simulink model "Fault_Estimator"  (R2023a)
settings: Solver=VariableStepAuto  StartTime=0.0  StopTime=60  RelTol=1e-3
values from neighbouring files (symbols this model uses):
  A = [O_As zeros(n,s)]    [Adaptive_Ka_Test.m]    (also in Fault_Estimator_Parameters.mat = [0.999941069129  7.16658673766e-07  5.87954926208e-05  0; -1; UIO_Calculation.m)
  A_bar = G*A    [Adaptive_Ka_Test.m]    (also in Fault_Estimator_Parameters.mat = [0 -1.34709716077e-07 5.89016941685e-05 -5.89016941685e-05 0; UIO_Calculation.m)
  A_zero = O_Az    [Adaptive_Ka_Test.m]    (also in Fault_Estimator_Parameters.mat = [0.00133629303608 -0.0295574271846 0.028990279103 0.00138410; LPV_Time_Varient_Parameter.m; UIO_Calculation.m)
  B = O_B    [Adaptive_Ka_Test.m]    (also in Fault_Estimator_Parameters.mat = [6.48267970563e-05  3.7353807763e-08; 6.66149393921e-09  6.4; LPV_Time_Varient_Parameter.m; UIO_Calculation.m)
  B_bar = G*B    [Adaptive_Ka_Test.m]    (also in Fault_Estimator_Parameters.mat = [0  0; 6.66149393921e-09  6.48911324748e-05; 6.63859792846e-; UIO_Calculation.m)
  C = [C_star F]    [Adaptive_Ka_Test.m]    (also in Fault_Estimator_Parameters.mat = [1  0  0  0; 0  1  0  0; 0  0  1  1]; UIO_Calculation.m)
  D = [1/154;0;0]    [Adaptive_Ka_Test.m]    (also in UIO_Calculation.m)
  E_zero = O_E*E    [Adaptive_Ka_Test.m]    (also in Fault_Estimator_Parameters.mat = [0.000413364504327 -0.000387576328554 -0.000192232694 -0.013; UIO_Calculation.m)
  G = T-T*D*H*C*T    [Adaptive_Ka_Test.m]    (also in Fault_Estimator_Parameters.mat = [0  0  0; 0  1  0; 0  0  1; 0  0  -1]; UIO_Calculation.m)
  H = inv(transpose(C*T*D)*C*T*D)*transpose(C*T*D)    [Adaptive_Ka_Test.m]    (also in Fault_Estimator_Parameters.mat = [154 0 0]; UIO_Calculation.m)
  Ka = inv(value(U))*value(N_bar)    [Adaptive_Ka_Test.m]    (also in Fault_Estimator_Parameters.mat = [-1.05152228748e-07  -0.00319474208396  -2.37139603589e-10; ; Ka.mat = [0.202280164209  0.202279756548  0.594992063891; 0.202157428; UIO_Calculation.m)
  L_bar = (N-T*D*H*C*N+T*D*H)    [Adaptive_Ka_Test.m]    (also in Fault_Estimator_Parameters.mat = [1  0  0; 0  0  0; 0  0  0; 0  0  1]; UIO_Calculation.m)
  N = temp(1:n+s,n+1:n+p)    [Adaptive_Ka_Test.m]    (also in Fault_Estimator_Parameters.mat = [0  0  0; 0  0  0; 0  0  0; 0  0  1]; UIO_Calculation.m)
  p = 3    [Adaptive_Ka_Test.m]    (also in Fault_Estimator_Parameters.mat; UIO_Calculation.m; test.m = plot(transpose(Xt_hat)-transpose(Xt(:,t+1:t+6000))))
  T = temp(1:n+s,1:n)    [Adaptive_Ka_Test.m]    (also in Fault_Estimator_Parameters.mat = [1  0  0; 0  1  0; 0  0  1; 0  0  -1]; UIO_Calculation.m)
libraries: simulink x2
settings Model: Creator=sepeh  LastModifiedBy=sepeh

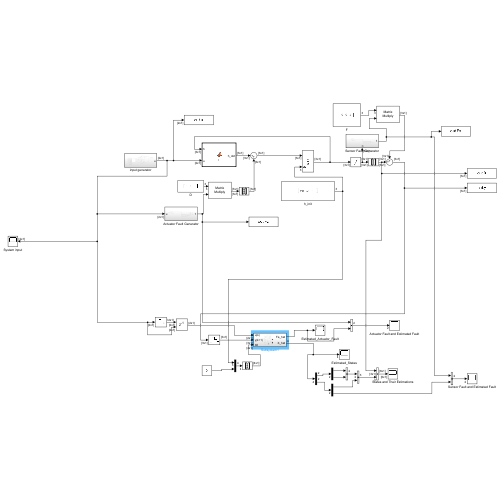
[thumbnail: Simulink's stored preview of the top-level diagram]
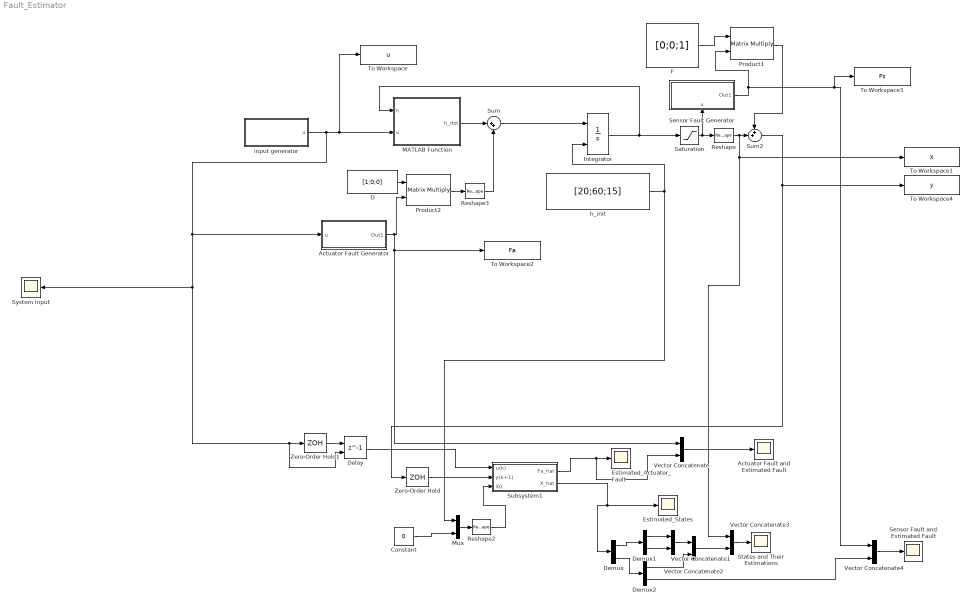
== system Fault_Estimator ==
  Actuator Fault Generator : Subsystem
  Actuator Fault and Estimated Fault : Scope
  Constant : Constant  Value=0
  D : Constant  Value=[1;0;0]
  Delay : Delay  DelayLength=1  InitialConditionSource=Input port  InitialCondition=0  SampleTime=0.01
      settings: InputPortMap=u0,p4
  Demux : Demux  Outputs=2
  Demux1 : Demux  Outputs=2
  Demux2 : Demux  Outputs=2
  Estimated_Actuator_Fault : Scope
  Estimated_States : Scope
  F : Constant  Value=[0;0;1]
  Integrator : Integrator  InitialConditionSource=external
  MATLAB Function : MATLAB Function  TreatAsAtomicUnit=on
  Mux : Mux  Inputs=2
  Product1 : Product  Multiplication=Matrix(*)
  Product2 : Product  Multiplication=Matrix(*)
  Reshape : Reshape  OutputDimensionality=Column vector (2-D)
  Reshape2 : Reshape  OutputDimensionality=Column vector (2-D)
  Reshape3 : Reshape  OutputDimensionality=Column vector (2-D)
  Saturation : Saturate  UpperLimit=100  LowerLimit=0
  Sensor Fault Generator : Subsystem
      settings: PortSchema="{\"entries\":[{\"content\":{\"sides\":[{\"content\":{},\"type\":\"ConnectorPlacement.EquallySpacedRectSide\",\"uuid\":\"8737017c-7270-4c54-a415-3a022d708922\"},{\"content\":{\"connectorIds\":[\"Out1\"],\"side\":\"RIGHT\"},\"type\":\"ConnectorPlacement.EquallySpacedRectSide\",\"uuid\":\"227575ae-1db5-4c8b-a626-16b54a509aa1\"},{\"content\":{\"side\":\"TOP\"},\"type\":\"ConnectorPlacement.EquallySpacedRectSide\",\"uuid\":\"ce2fa024-2e15-4882-8a20-94458726743e\"},{\"content\":{\"connectorIds\":[\"In1\"],\"side\":\"BOTTOM\"},\"type\":\"ConnectorPlacement.EquallySpacedRectSide\",\"uuid\":\"c4ae589d-782a-4398-85fd-5b05ba97c294\"}]},\"type\":\"ConnectorPlacement.EquallySpacedConnector\",\"uuid\":\"70d82ebf-b199-4a7a-86b9-c10264c6c64d\"}],\"packageUris\":[\"http://schema.mathworks.com/mf0/Connector/R2020b\"],\"version\":\"1.0\"}"
  Sensor Fault and Estimated Fault : Scope
  States and Their Estimations : Scope
  Subsystem1 : Subsystem
  Sum : Sum  Inputs=|++
  Sum2 : Sum  Inputs=++|
  System input : Scope
  To Workspace : ToWorkspace  VariableName=u  SaveFormat=Timeseries  SampleTime=0.01
  To Workspace1 : ToWorkspace  VariableName=X  SaveFormat=Timeseries  SampleTime=0.01
  To Workspace2 : ToWorkspace  VariableName=Fa  SaveFormat=Timeseries  SampleTime=0.01
  To Workspace3 : ToWorkspace  VariableName=Fs  SaveFormat=Timeseries  SampleTime=0.01
  To Workspace4 : ToWorkspace  VariableName=y  SaveFormat=Timeseries  SampleTime=0.01
  Vector Concatenate{,1..4} (5 alike) : Concatenate
  Zero-Order Hold : ZeroOrderHold  SampleTime=0.01
  Zero-Order Hold1 : ZeroOrderHold  SampleTime=0.01
  h_init : Constant  Value=[20;60;15]
  input generator : Subsystem
  wires:
  Integrator/1 -> Saturation/1, MATLAB Function/1(h)
  Zero-Order Hold1/1 -> Delay/1
  Delay/1 -> Subsystem1/1(u(k))
  Zero-Order Hold/1 -> Subsystem1/2(y(k+1))
  Sum2/1 -> To Workspace4/1, Zero-Order Hold/1
  input generator/1(u) -> To Workspace/1, MATLAB Function/2(u), Actuator Fault Generator/1(u), Delay/2, Zero-Order Hold1/1, System input/1
  MATLAB Function/1(h_dot) -> Sum/1
  Sum/1 -> Integrator/1
  Subsystem1/2(X_hat) -> Estimated_States/1, Demux/1
  Subsystem1/1(Fa_hat) -> Vector Concatenate/2, Estimated_Actuator_Fault/1
  Vector Concatenate/1 -> Actuator Fault and Estimated Fault/1
  h_init/1 -> Mux/1, Integrator/2
  F/1 -> Product1/1
  Saturation/1 -> Reshape/1, Sensor Fault Generator/1(u)
  Reshape/1 -> To Workspace1/1, Vector Concatenate3/1, Sum2/2
  Product1/1 -> Sum2/1
  Constant/1 -> Mux/2
  Mux/1 -> Reshape2/1
  Reshape2/1 -> Subsystem1/3(X0)
  D/1 -> Product2/1
  Reshape3/1 -> Sum/2
  Product2/1 -> Reshape3/1
  Demux/1 -> Demux1/1
  Demux/2 -> Demux2/1
  Demux1/1 -> Vector Concatenate1/1
  Demux1/2 -> Vector Concatenate1/2
  Vector Concatenate1/1 -> Vector Concatenate2/1
  Demux2/1 -> Vector Concatenate2/2
  Vector Concatenate2/1 -> Vector Concatenate3/2
  Vector Concatenate3/1 -> States and Their Estimations/1
  Demux2/2 -> Vector Concatenate4/2
  Actuator Fault Generator/1(Out1) -> To Workspace2/1, Vector Concatenate/1, Product2/2
  Vector Concatenate4/1 -> Sensor Fault and Estimated Fault/1
  Sensor Fault Generator/1(Out1) -> Product1/2, To Workspace3/1, Vector Concatenate4/1

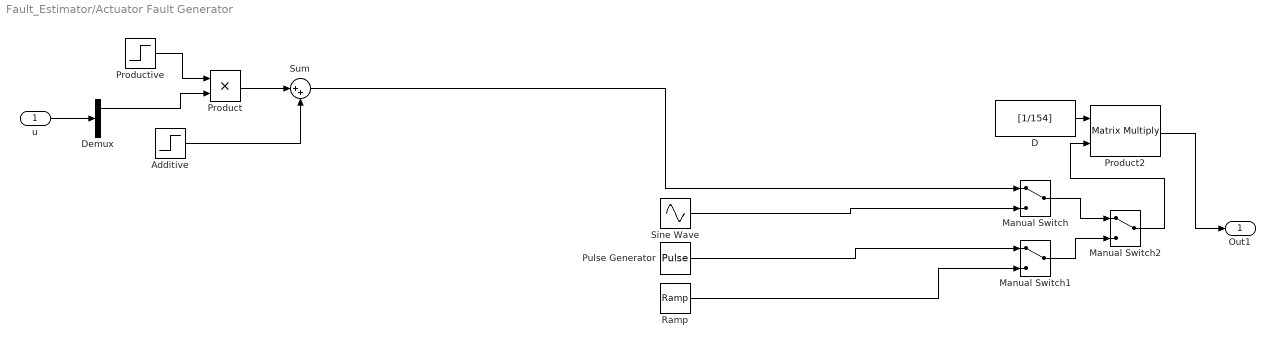
== system Fault_Estimator/Actuator Fault Generator ==
  u : Inport
  Additive : Step  Time=20  After=-10  SampleTime=0
  D : Constant  Value=[1/154]
  Demux : Demux  Outputs=2
  Manual Switch : ManualSwitch
  Manual Switch1 : ManualSwitch
  Manual Switch2 : ManualSwitch
  Product : Product
  Product2 : Product  Multiplication=Matrix(*)
  Productive : Step  Time=20  After=-0.2  SampleTime=0
  Pulse Generator : DiscretePulseGenerator  PulseType=Time based  Amplitude=-100  Period=10  PulseWidth=50
  Ramp : simulink/Sources/Ramp  slope=-10  start=30  InitialOutput=0
  Sine Wave : Sin  Amplitude=50  Bias=-100  SampleTime=0
  Sum : Sum  Inputs=|++
  Out1 : Outport
  wires:
  Manual Switch1/1 -> Manual Switch2/2
  Manual Switch/1 -> Manual Switch2/1
  u/1 -> Demux/1
  Demux/1 -> Product/2
  Product/1 -> Sum/1
  Sum/1 -> Manual Switch/1
  Additive/1 -> Sum/2
  Productive/1 -> Product/1
  Sine Wave/1 -> Manual Switch/2
  Pulse Generator/1 -> Manual Switch1/1
  Ramp/1 -> Manual Switch1/2
  D/1 -> Product2/1
  Manual Switch2/1 -> Product2/2
  Product2/1 -> Out1/1

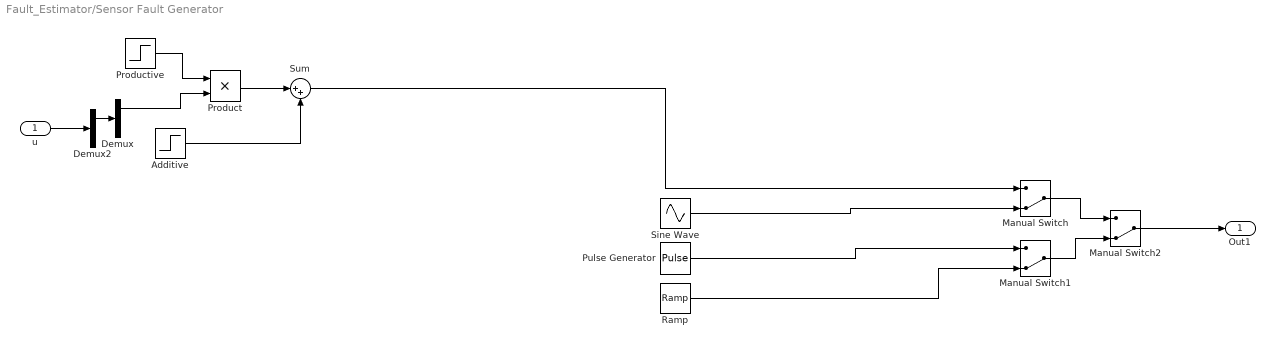
== system Fault_Estimator/Sensor Fault Generator ==
  u : Inport
  Additive : Step  Time=20  After=-10  SampleTime=0
  Demux : Demux  Outputs=2
  Demux2 : Demux  Outputs=2
  Manual Switch : ManualSwitch  CurrentSetting=0
  Manual Switch1 : ManualSwitch  CurrentSetting=0
  Manual Switch2 : ManualSwitch  CurrentSetting=0
  Product : Product
  Productive : Step  Time=20  After=-0.2  SampleTime=0
  Pulse Generator : DiscretePulseGenerator  PulseType=Time based  Amplitude=-20  Period=10  PulseWidth=50
  Ramp : simulink/Sources/Ramp  slope=-1  start=30  InitialOutput=0
  Sine Wave : Sin  Amplitude=50  Bias=-100  SampleTime=0
  Sum : Sum  Inputs=|++
  Out1 : Outport
  wires:
  Manual Switch1/1 -> Manual Switch2/2
  Manual Switch/1 -> Manual Switch2/1
  Manual Switch2/1 -> Out1/1
  Demux/1 -> Product/2
  Product/1 -> Sum/1
  Sum/1 -> Manual Switch/1
  Additive/1 -> Sum/2
  Productive/1 -> Product/1
  Sine Wave/1 -> Manual Switch/2
  Pulse Generator/1 -> Manual Switch1/1
  Ramp/1 -> Manual Switch1/2
  Demux2/1 -> Demux/1
  u/1 -> Demux2/1

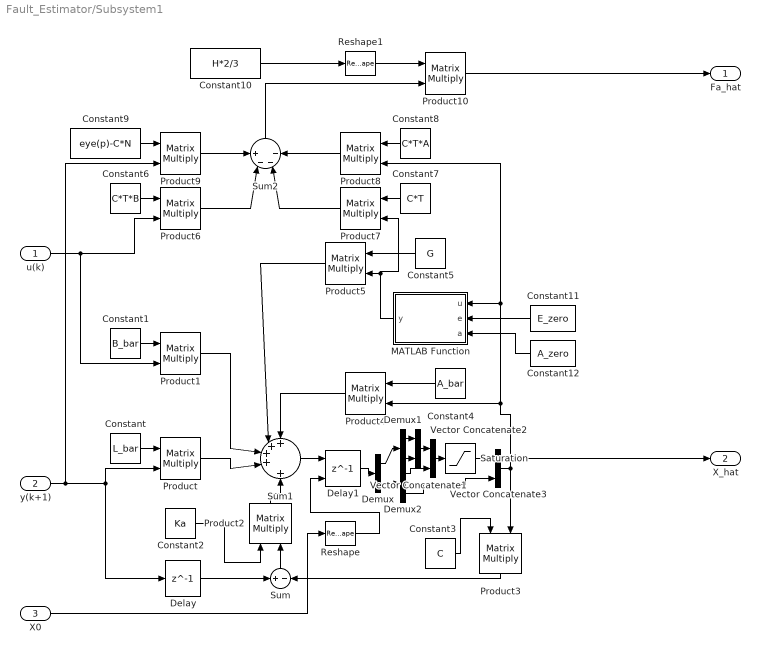
== system Fault_Estimator/Subsystem1 ==
  u(k) : Inport
  y(k+1) : Inport  Port=2
  X0 : Inport  Port=3
  Constant : Constant  Value=L_bar
  Constant1 : Constant  Value=B_bar
  Constant10 : Constant  Value=H*2/3
  Constant11 : Constant  Value=E_zero
  Constant12 : Constant  Value=A_zero
  Constant2 : Constant  Value=Ka
  Constant3 : Constant  Value=C
  Constant4 : Constant  Value=A_bar
  Constant5 : Constant  Value=G
  Constant6 : Constant  Value=C*T*B
  Constant7 : Constant  Value=C*T
  Constant8 : Constant  Value=C*T*A
  Constant9 : Constant  Value=eye(p)-C*N
  Delay : Delay  DelayLength=1  InitialCondition=[0;0;0]
  Delay1 : Delay  DelayLength=1  InitialConditionSource=Input port  InitialCondition=[0;0;0]
      settings: InputPortMap=u0,p4
  Demux : Demux  Outputs=2
  Demux1 : Demux  Outputs=2
  Demux2 : Demux  Outputs=2
  MATLAB Function : MATLAB Function  TreatAsAtomicUnit=on
  Product{,1..10} (11 alike) : Product  Multiplication=Matrix(*)
  Reshape : Reshape  OutputDimensionality=Column vector (2-D)
  Reshape1 : Reshape  OutputDimensionality=Row vector (2-D)
  Saturation : Saturate  UpperLimit=100  LowerLimit=0
  Sum : Sum  Inputs=+|-
  Sum1 : Sum  Inputs=++++|+
  Sum2 : Sum  Inputs=+---
  Vector Concatenate1 : Concatenate
  Vector Concatenate2 : Concatenate
  Vector Concatenate3 : Concatenate
  Fa_hat : Outport
  X_hat : Outport  Port=2
  wires:
  Constant/1 -> Product/1
  Constant1/1 -> Product1/1
  Delay/1 -> Sum/1
  Sum/1 -> Product2/2
  Constant2/1 -> Product2/1
  Product2/1 -> Sum1/5
  Product/1 -> Sum1/4
  Product1/1 -> Sum1/3
  Sum1/1 -> Delay1/1
  Vector Concatenate3/1 -> Product3/2, X_hat/1, Product8/2, MATLAB Function/1(u), Product4/2
  Product3/1 -> Sum/2
  Constant3/1 -> Product3/1
  Constant4/1 -> Product4/1
  Product4/1 -> Sum1/1
  Constant5/1 -> Product5/1
  MATLAB Function/1(y) -> Product7/2, Product5/2
  Product5/1 -> Sum1/2
  Constant6/1 -> Product6/1
  u(k)/1 -> Product1/2, Product6/2
  Constant7/1 -> Product7/1
  Constant8/1 -> Product8/1
  Constant9/1 -> Product9/1
  Product9/1 -> Sum2/1
  Product8/1 -> Sum2/4
  Product6/1 -> Sum2/2
  Product7/1 -> Sum2/3
  Product10/1 -> Fa_hat/1
  Sum2/1 -> Product10/2
  Constant11/1 -> MATLAB Function/2(e)
  Constant12/1 -> MATLAB Function/3(a)
  y(k+1)/1 -> Delay/1, Product/2, Product9/2
  X0/1 -> Reshape/1
  Reshape/1 -> Delay1/2
  Constant10/1 -> Reshape1/1
  Reshape1/1 -> Product10/1
  Demux/2 -> Demux2/1
  Demux1/1 -> Vector Concatenate1/1
  Demux1/2 -> Vector Concatenate1/2
  Demux/1 -> Demux1/1
  Vector Concatenate1/1 -> Vector Concatenate2/1
  Demux2/1 -> Vector Concatenate2/2
  Vector Concatenate2/1 -> Saturation/1
  Demux2/2 -> Vector Concatenate3/2
  Delay1/1 -> Demux/1
  Saturation/1 -> Vector Concatenate3/1

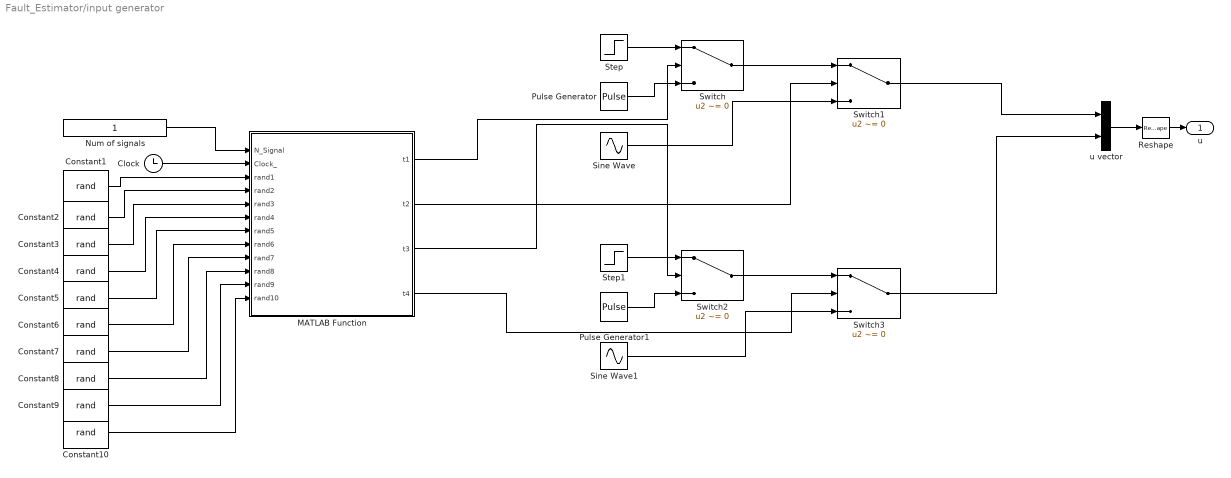
== system Fault_Estimator/input generator ==
  Clock : Clock
  Constant{1..10} (10 alike) : Constant  Value=rand
  MATLAB Function : MATLAB Function  TreatAsAtomicUnit=on
  Num of signals : Constant
  Pulse Generator : DiscretePulseGenerator  PulseType=Time based  Amplitude=rand*250  Period=rand*60  PulseWidth=rand*100
  Pulse Generator1 : DiscretePulseGenerator  PulseType=Time based  Amplitude=rand*250  Period=rand*60  PulseWidth=rand*100
  Reshape : Reshape  OutputDimensionality=Column vector (2-D)
  Sine Wave : Sin  Amplitude=rand*125  Bias=125  Frequency=((pi)-1.053e-01)*rand + 1.053e-01  SampleTime=0
  Sine Wave1 : Sin  Amplitude=rand*125  Bias=125  Frequency=((pi)-1.053e-01)*rand + 1.053e-01  SampleTime=0
  Step : Step  Time=rand*60  After=rand*250  SampleTime=0
  Step1 : Step  Time=rand*60  After=rand*250  SampleTime=0
  Switch{,1..3} (4 alike) : Switch  Criteria=u2 ~= 0  Threshold=rand*300  SaturateOnIntegerOverflow=off  InputSameDT=off
  u vector : Concatenate
  u : Outport
  wires:
  u vector/1 -> Reshape/1
  Reshape/1 -> u/1
  Switch1/1 -> u vector/1
  Switch3/1 -> u vector/2
  Pulse Generator/1 -> Switch/3
  Switch2/1 -> Switch3/1
  Switch/1 -> Switch1/1
  Pulse Generator1/1 -> Switch2/3
  Step/1 -> Switch/1
  Step1/1 -> Switch2/1
  Sine Wave1/1 -> Switch3/3
  Sine Wave/1 -> Switch1/3
  MATLAB Function/1(t1) -> Switch/2
  MATLAB Function/2(t2) -> Switch1/2
  MATLAB Function/3(t3) -> Switch2/2
  MATLAB Function/4(t4) -> Switch3/2
  Clock/1 -> MATLAB Function/2(Clock_)
  Num of signals/1 -> MATLAB Function/1(N_Signal)
  Constant1/1 -> MATLAB Function/3(rand1)
  Constant2/1 -> MATLAB Function/4(rand2)
  Constant3/1 -> MATLAB Function/5(rand3)
  Constant4/1 -> MATLAB Function/6(rand4)
  Constant5/1 -> MATLAB Function/7(rand5)
  Constant6/1 -> MATLAB Function/8(rand6)
  Constant7/1 -> MATLAB Function/9(rand7)
  Constant8/1 -> MATLAB Function/10(rand8)
  Constant9/1 -> MATLAB Function/11(rand9)
  Constant10/1 -> MATLAB Function/12(rand10)

== matlab function Fault_Estimator/input generator/MATLAB Function ==
  data: t1 output; t2 output; t3 output; t4 output; N_Signal input; Clock_ input; rand1 input; rand2 input; rand3 input; rand4 input; rand5 input; rand6 input; rand7 input; rand8 input; rand9 input; rand10 input
function [t1,t2,t3,t4]= time_manager(N_Signal,Clock_,rand1,rand2,rand3,rand4,rand5,rand6,rand7,rand8,rand9,rand10)
t1=0;
t2=0;
t3=0;
t4=0;
period=60;
if N_Signal<=1
    [t1,t2]=Switch_selector(rand1*3);
    [t3,t4]=Switch_selector(rand2*3);
elseif N_Signal<=2
    change_time1=rand1*period;
    if(change_time1>=Clock_)
        [t1,t2]=Switch_selector(rand2*3);
    else
        [t1,t2]=Switch_selector(rand3*3);
    end
    change_time2=rand2*period;
    if(change_time2>=Clock_)
        [t3,t4]=Switch_selector(rand4*3);
    else
        [t3,t4]=Switch_selector(rand5*3);
    end
else
    change_time_1_1=rand1*period;
    change_time_1_2=(period-change_time_1_1)*rand2+change_time_1_1;
    change_time_2_1=rand3*period;
    change_time_2_2=(period-change_time_2_1)*rand4+change_time_2_1;
    if change_time_1_1>Clock_
        [t1,t2]=Switch_selector(rand5*3);
    elseif change_time_1_1<=Clock_ && change_time_1_2>=Clock_
        [t1,t2]=Switch_selector(rand6*3);
    elseif change_time_1_2<Clock_
        [t1,t2]=Switch_selector(rand7*3);
    end
    if change_time_2_1>Clock_
        [t3,t4]=Switch_selector(rand8*3);
    elseif change_time_2_1<=Clock_ && change_time_2_2>=Clock_
        [t3,t4]=Switch_selector(rand9*3);
    elseif change_time_2_2<Clock_
        [t3,t4]=Switch_selector(rand10*3);
    end
end

== matlab function Fault_Estimator/MATLAB Function ==
  data: h input; u input; h_dot output
function h_dot = f(h,u)
g=1000;
A=154;
a1=0.46;
a2=0.6;
a3=0.45;
S13=0.5;
S23=0.5;
S2o=0.5;
Q13=a1*S13*sign(h(1)-h(3))*sqrt(2*g*abs(h(1)-h(3)));
Q23=a3*S23*sign(h(3)-h(2))*sqrt(2*g*abs(h(3)-h(2)));
Q2o=a2*S2o*sqrt(abs(2*g*h(2)));
h_dot = 1/A*[u(1)-Q13;u(2)+Q23-Q2o;Q13-Q23];

== matlab function Fault_Estimator/Subsystem1/MATLAB Function ==
  data: u input; y output; e input; a input
function y = fcn(u,e,a)

y = a*(tanh(e*u));
